simulink model "UCIe_Model"  (R2024a)
settings: Solver=VariableStepAuto  StartTime=0.0  StopTime=10.0  RelTol=1e-3
libraries: commchan3 x1, commsink2 x1
settings Model: Creator=dhirajkrishnasimhadri  LastModifiedBy=dhirajkrishnasimhadri

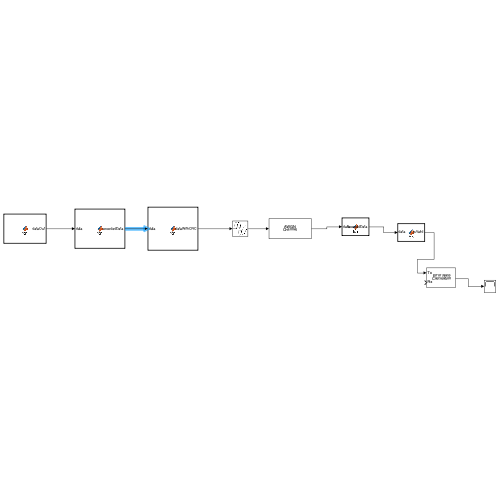
[thumbnail: Simulink's stored preview of the top-level diagram]
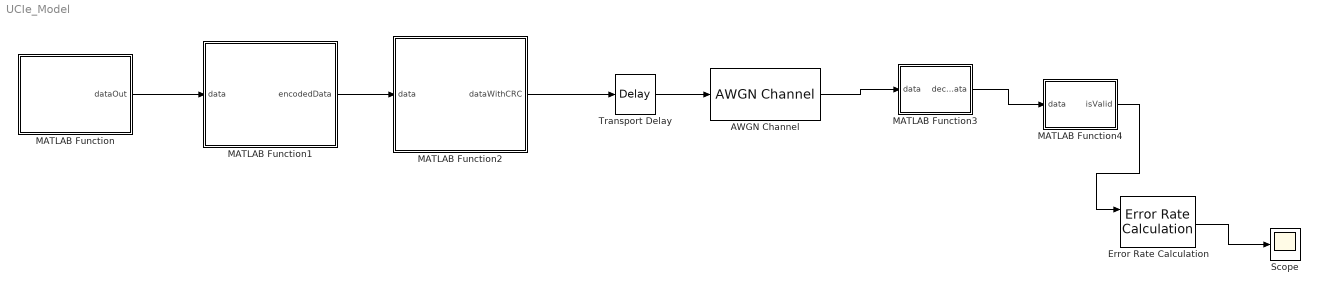
== system UCIe_Model ==
  AWGN Channel : commchan3/AWGN Channel  LegacyMode=off  NoiseMethod="Signal to noise ratio  (Eb/No)"  noiseMode="Signal to noise ratio  (SNR)"  EbNo=10  EsNo=10  SNR=10  BitsPerSymbol=1  SignalPower=1  SamplesPerSymbol=1  SymbolPeriod=1  VarianceSource=Parameter  Variance=1  RandomStream=Global stream  Seed=67  SimulateUsing=Code generation
  Error Rate Calculation : commsink2/Error Rate Calculation  N=0  st_delay=0  cp_mode=Entire frame  subframe=[]  PMode=Port  WsName=ErrorVec  RsMode2=off  stop=off  numErr=100  maxBits=1e6
  MATLAB Function : MATLAB Function  TreatAsAtomicUnit=on
  MATLAB Function1 : MATLAB Function  TreatAsAtomicUnit=on
  MATLAB Function2 : MATLAB Function  TreatAsAtomicUnit=on
  MATLAB Function3 : MATLAB Function  TreatAsAtomicUnit=on
  MATLAB Function4 : MATLAB Function  TreatAsAtomicUnit=on
  Scope : Scope
  Transport Delay : TransportDelay  DelayTime=1.2e-9
  wires:
  MATLAB Function/1(dataOut) -> MATLAB Function1/1(data)
  MATLAB Function1/1(encodedData) -> MATLAB Function2/1(data)
  MATLAB Function2/1(dataWithCRC) -> Transport Delay/1
  Transport Delay/1 -> AWGN Channel/1
  AWGN Channel/1 -> MATLAB Function3/1(data)
  MATLAB Function3/1(decodedData) -> MATLAB Function4/1(data)
  MATLAB Function4/1(isValid) -> Error Rate Calculation/1
  Error Rate Calculation/1 -> Scope/1

== matlab function UCIe_Model/MATLAB Function ==
  data: dataOut output
function dataOut = fcn()
    dataOut = generateData(8000); % Generate 8000 bits
end

== matlab function UCIe_Model/MATLAB Function2 ==
  data: data input; dataWithCRC output
function dataWithCRC = fcn(data)
    dataWithCRC = addCRC(data);
end

== matlab function UCIe_Model/MATLAB Function3 ==
  data: data input; decodedData output
function decodedData = fcn(data)
    decodedData = decode8b10b(data);
end

== matlab function UCIe_Model/MATLAB Function4 ==
  data: data input; isValid output
function isValid = fcn(data)
    isValid = checkCRC(data);
end

== matlab function UCIe_Model/MATLAB Function1 ==
  data: data input; encodedData output
function encodedData = fcn(data)
    encodedData = encode8b10b(data);
end
